simulink model "cascaded3lvl"  (R2023b)
settings: Solver=ode4  StartTime=0.0  StopTime=0.1  FixedStep=1e-5  RelTol=1e-3
libraries: spsIGBTDiodeLib x12, simulink x6, spsDCVoltageSourceLib x3, spsSeriesRLCBranchLib x3, spsGroundLib x2, spsThreePhaseVIMeasurementLib x1, sps_lib x1
settings Model: Creator=user  LastModifiedBy=user

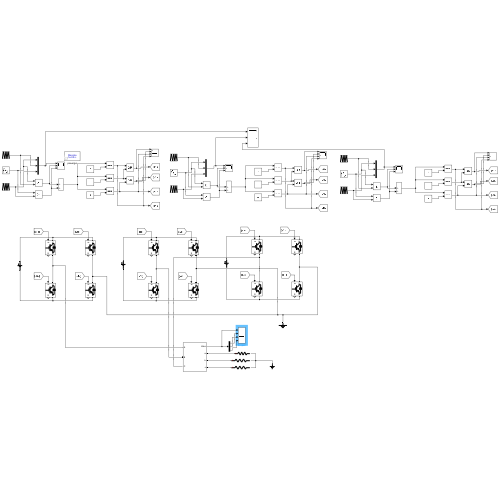
[thumbnail: Simulink's stored preview of the top-level diagram]
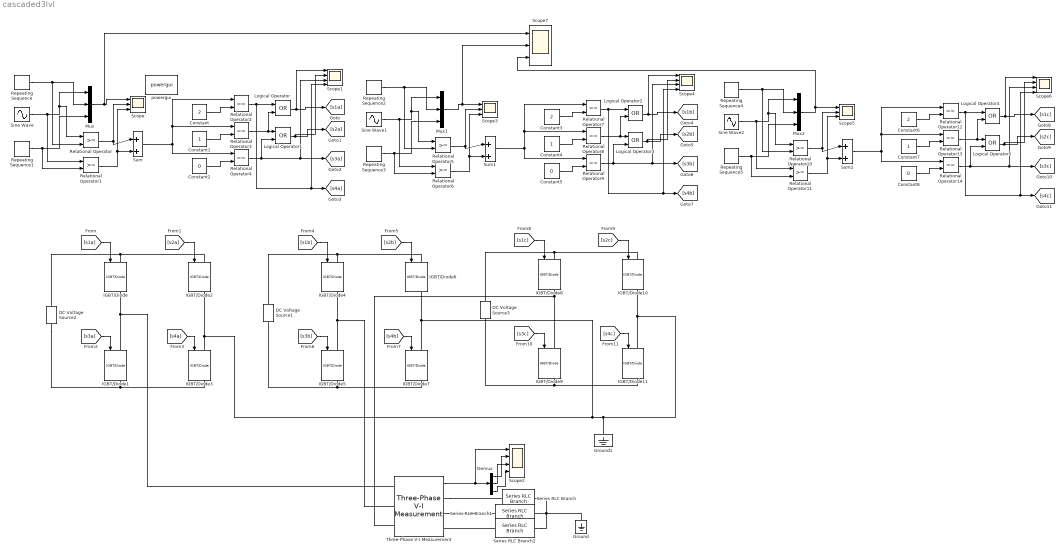
== system cascaded3lvl ==
  Constant : Constant  Value=2
  Constant1 : Constant
  Constant2 : Constant  Value=0
  Constant3 : Constant  Value=2
  Constant4 : Constant
  Constant5 : Constant  Value=0
  Constant6 : Constant  Value=2
  Constant7 : Constant
  Constant8 : Constant  Value=0
  DC Voltage Source1 : spsDCVoltageSourceLib/DC Voltage Source  Amplitude=100  Measurements=None
  DC Voltage Source2 : spsDCVoltageSourceLib/DC Voltage Source  Amplitude=100  Measurements=None
  DC Voltage Source3 : spsDCVoltageSourceLib/DC Voltage Source  Amplitude=100  Measurements=None
  Demux : Demux  Outputs=3
  Ground : spsGroundLib/Ground  LConnTagsString=a
  Ground1 : spsGroundLib/Ground  LConnTagsString=a
  IGBT/Diode{,1..11} (12 alike) : spsIGBTDiodeLib/IGBT//Diode  Ron=1e-3  Rs=1e5  Cs=inf  Measurements=on
  Logical Operator{,1..5} (6 alike) : Logic  Operator=OR  AllPortsSameDT=off  OutDataTypeStr=boolean
  Mux : Mux  Inputs=3
  Mux1 : Mux  Inputs=3
  Mux2 : Mux  Inputs=3
  Relational Operator{,1,5..6,10..11} (6 alike) : RelationalOperator  OutDataTypeStr=boolean  RndMeth=Simplest  InputSameDT=off
  Relational Operator{2..4,7..9,12..14} (9 alike) : RelationalOperator  Operator===  OutDataTypeStr=boolean  RndMeth=Simplest  InputSameDT=off
  Repeating Sequence : simulink/Sources/Repeating Sequence  rep_seq_t=[0 1 2]*[1/400]  rep_seq_y=[0 1 0]
  Repeating Sequence1 : simulink/Sources/Repeating Sequence  rep_seq_t=[0 1 2]*[1/400]  rep_seq_y=[-1 0 -1]
  Repeating Sequence2 : simulink/Sources/Repeating Sequence  rep_seq_t=[0 1 2]*[1/400]  rep_seq_y=[0 1 0]
  Repeating Sequence3 : simulink/Sources/Repeating Sequence  rep_seq_t=[0 1 2]*[1/400]  rep_seq_y=[-1 0 -1]
  Repeating Sequence4 : simulink/Sources/Repeating Sequence  rep_seq_t=[0 1 2]*[1/400]  rep_seq_y=[0 1 0]
  Repeating Sequence5 : simulink/Sources/Repeating Sequence  rep_seq_t=[0 1 2]*[1/400]  rep_seq_y=[-1 0 -1]
  Scope{,3,5,7} (4 alike) : Scope  NumInputPorts=3
  Scope{1..2,4,6} (4 alike) : Scope  NumInputPorts=4
  Series RLC Branch : spsSeriesRLCBranchLib/Series RLC Branch  LConnTagsString=__new0  RConnTagsString=__new0  BranchType=R  Resistance=500  Inductance=1e-3  SetiL0=off  InitialCurrent=0  Capacitance=1e-6  Setx0=off  InitialVoltage=0  Measurements=Branch voltage
  Series RLC Branch1 : spsSeriesRLCBranchLib/Series RLC Branch  LConnTagsString=__new0  RConnTagsString=__new0  BranchType=R  Resistance=100  Inductance=1e-3  SetiL0=off  InitialCurrent=0  Capacitance=1e-6  Setx0=off  InitialVoltage=0  Measurements=Branch voltage
  Series RLC Branch2 : spsSeriesRLCBranchLib/Series RLC Branch  LConnTagsString=__new0  RConnTagsString=__new0  BranchType=R  Resistance=250  Inductance=1e-3  SetiL0=off  InitialCurrent=0  Capacitance=1e-6  Setx0=off  InitialVoltage=0  Measurements=Branch voltage
  Sine Wave : Sin  Frequency=2*pi*50  SampleTime=0
  Sine Wave1 : Sin  Frequency=2*pi*50  Phase=4*pi/3  SampleTime=0
  Sine Wave2 : Sin  Frequency=2*pi*50  Phase=2*pi/3  SampleTime=0
  Sum : Sum  Inputs=|++
  Sum1 : Sum  Inputs=|++
  Sum2 : Sum  Inputs=|++
  Three-Phase V-I Measurement : spsThreePhaseVIMeasurementLib/Three-Phase V-I Measurement  VoltageMeasurement=phase-to-ground  SetLabelV=off  LabelV=Vabc  Vpu=off  VpuLL=off  CurrentMeasurement=no  SetLabelI=off  LabelI=Iabc  Ipu=off  Pbase=100e6  Vbase=500e3  OutputType=Complex  PhasorSimulation=off  PSBequivalent=0
  powergui : sps_lib/powergui  Priority=1  SimulationMode=Discrete  SampleTime=1e-5  frequency=60  Iterations=50  frequencyindice=0  Pbase=100e6  ErrMax=1e-4  UnitsV=kV  UnitsW=MW  buscounter=0  FunctionMessages=off  echomessages=off  EnableUseOfTLC=off  CurrentSourceSwitches=off  DisableSnubberDevices=off  DisableRonSwitches=off  DisableVfSwitches=off  DisplayEquations=off  AutomaticDiscreteSolvers=off  SolverType=Tustin  Interpol=off  ExternalGateDelay=off  methode=off  Ts=0  x0status=blocks  SPID=off  SwTol=0  HookPort=off  NonlinearTolerance=1e-4  nMaxIteration=100  ContinueOnMaxIteration=off  RestoreLinks=warning  ResistiveCurrentMeasurement=off  Frange=[0:2:500]  Ylog=off  Xlog=on  ShowGrid=off  save=off  variable=ZData  structure=ScopeData  ZoomFFT=off  StartTime=0.02  cycles=1  DisplayStyle=1  fundamental=50  FreqAxis=off  MaxFrequency=1000  frequencyindicesteady=1  RmsSteady=1  display=off
  wires:
  Sine Wave/1 -> Relational Operator1/1, Mux/1, Relational Operator/1
  Repeating Sequence/1 -> Relational Operator/2, Mux/2
  Repeating Sequence1/1 -> Relational Operator1/2, Mux/3
  Relational Operator/1 -> Scope/2, Sum/1
  Relational Operator1/1 -> Sum/2, Scope/3
  Sum/1 -> Relational Operator4/1, Relational Operator3/1, Relational Operator2/1
  Constant/1 -> Relational Operator2/2
  Constant1/1 -> Relational Operator3/2
  Constant2/1 -> Relational Operator4/2
  Relational Operator2/1 -> Scope1/4, [s4a], Logical Operator/1
  Relational Operator3/1 -> Logical Operator1/1, Logical Operator/2
  Relational Operator4/1 -> Logical Operator1/2, Scope1/3, [s3a]
  Logical Operator1/1 -> Scope1/2, [s2a]
  Logical Operator/1 -> Scope1/1, [s1a]
  [s1a] -> IGBT/Diode/1
  [s3a] -> IGBT/Diode1/1
  [s2a] -> IGBT/Diode2/1
  [s4a] -> IGBT/Diode3/1
  Constant3/1 -> Relational Operator7/2
  Relational Operator8/1 -> Logical Operator3/1, Logical Operator2/2
  Constant4/1 -> Relational Operator8/2
  Relational Operator7/1 -> Scope4/4, [s4b], Logical Operator2/1
  Sine Wave1/1 -> Relational Operator6/1, Mux1/1, Relational Operator5/1
  Constant5/1 -> Relational Operator9/2
  Logical Operator2/1 -> Scope4/1, [s1b]
  Logical Operator3/1 -> Scope4/2, [s2b]
  Sum1/1 -> Relational Operator9/1, Relational Operator8/1, Relational Operator7/1
  Relational Operator9/1 -> Logical Operator3/2, Scope4/3, [s3b]
  Mux1/1 -> Scope7/2, Scope3/1
  Relational Operator6/1 -> Sum1/2, Scope3/3
  Repeating Sequence3/1 -> Relational Operator6/2, Mux1/3
  Repeating Sequence2/1 -> Relational Operator5/2, Mux1/2
  Relational Operator5/1 -> Scope3/2, Sum1/1
  Constant6/1 -> Relational Operator12/2
  Relational Operator13/1 -> Logical Operator5/1, Logical Operator4/2
  Constant7/1 -> Relational Operator13/2
  Relational Operator12/1 -> Scope6/4, [s4c], Logical Operator4/1
  Sine Wave2/1 -> Relational Operator11/1, Mux2/1, Relational Operator10/1
  Constant8/1 -> Relational Operator14/2
  Logical Operator4/1 -> Scope6/1, [s1c]
  Logical Operator5/1 -> Scope6/2, [s2c]
  Sum2/1 -> Relational Operator14/1, Relational Operator13/1, Relational Operator12/1
  Relational Operator14/1 -> Logical Operator5/2, Scope6/3, [s3c]
  Mux2/1 -> Scope7/3, Scope5/1
  Relational Operator11/1 -> Sum2/2, Scope5/3
  Repeating Sequence5/1 -> Relational Operator11/2, Mux2/3
  Repeating Sequence4/1 -> Relational Operator10/2, Mux2/2
  Relational Operator10/1 -> Scope5/2, Sum2/1
  [s1b] -> IGBT/Diode4/1
  [s2b] -> IGBT/Diode6/1
  [s3b] -> IGBT/Diode5/1
  [s4b] -> IGBT/Diode7/1
  [s1c] -> IGBT/Diode8/1
  [s2c] -> IGBT/Diode10/1
  [s3c] -> IGBT/Diode9/1
  [s4c] -> IGBT/Diode11/1
  Three-Phase V-I Measurement/1 -> Scope2/1, Demux/1
  Demux/1 -> Scope2/2
  Demux/2 -> Scope2/3
  Demux/3 -> Scope2/4
  Mux/1 -> Scope7/1, Scope/1
  connections:
  DC Voltage Source2/RConn1 -- IGBT/Diode2/LConn1 -- IGBT/Diode/LConn1
  DC Voltage Source2/LConn1 -- IGBT/Diode3/RConn1 -- IGBT/Diode1/RConn1
  IGBT/Diode1/LConn1 -- Three-Phase V-I Measurement/LConn1 -- IGBT/Diode/RConn1
  IGBT/Diode4/LConn1 -- DC Voltage Source1/RConn1 -- IGBT/Diode6/LConn1
  IGBT/Diode5/RConn1 -- DC Voltage Source1/LConn1 -- IGBT/Diode7/RConn1
  IGBT/Diode5/LConn1 -- Three-Phase V-I Measurement/LConn2 -- IGBT/Diode4/RConn1
  IGBT/Diode8/LConn1 -- DC Voltage Source3/RConn1 -- IGBT/Diode10/LConn1
  IGBT/Diode9/RConn1 -- DC Voltage Source3/LConn1 -- IGBT/Diode11/RConn1
  IGBT/Diode9/LConn1 -- Three-Phase V-I Measurement/LConn3 -- IGBT/Diode8/RConn1
  IGBT/Diode3/LConn1 -- Ground1/LConn1 -- IGBT/Diode11/LConn1 -- IGBT/Diode10/RConn1 -- IGBT/Diode7/LConn1 -- IGBT/Diode6/RConn1 -- IGBT/Diode2/RConn1
  Series RLC Branch2/LConn1 -- Three-Phase V-I Measurement/RConn3
  Three-Phase V-I Measurement/RConn2 -- Series RLC Branch1/LConn1
  Three-Phase V-I Measurement/RConn1 -- Series RLC Branch/LConn1
  Series RLC Branch/RConn1 -- Ground/LConn1 -- Series RLC Branch2/RConn1 -- Series RLC Branch1/RConn1
